simulink model "Modello_lineare_Hinfsyn"  (R2022b)
settings: Solver=VariableStepAuto  StartTime=0.0  StopTime=60  RelTol=1e-3
values from neighbouring files (symbols this model uses):
  A_tot = [A_nom B_nom*C_att ... (first row only)    [Inizializzazione_segway.m]    (also in LQG_controller.m = load("Matrici spazio di stato.mat","A_tot").A_tot; Matrici spazio di stato.mat = [0 79.8818966561 0 0 1 0 0 0 0 -0.384250591166 -200 0 ... (1)
  B_tot = [zeros(2,2); B_att]    [Inizializzazione_segway.m]    (also in LQG_controller.m = load("Matrici spazio di stato.mat","B_tot").B_tot; Matrici spazio di stato.mat = [0  0; 0  0; 894.427191  0; 0  894.427191])
  C_tot = [C_nom zeros(2,2)]    [Inizializzazione_segway.m]    (also in LQG_controller.m = load("Matrici spazio di stato.mat","C_tot").C_tot; Matrici spazio di stato.mat = [1  0  0  0; 0  1  0  0])
  D_tot = zeros(2,2)    [Inizializzazione_segway.m]    (also in LQG_controller.m = load("Matrici spazio di stato.mat","D_tot").D_tot; Matrici spazio di stato.mat = [0  0; 0  0])
undefined symbols (not defined in the file or in its folder): K_ms, K_musyn
libraries: simulink x2
settings Model: Creator=anton  LastModifiedBy=angel

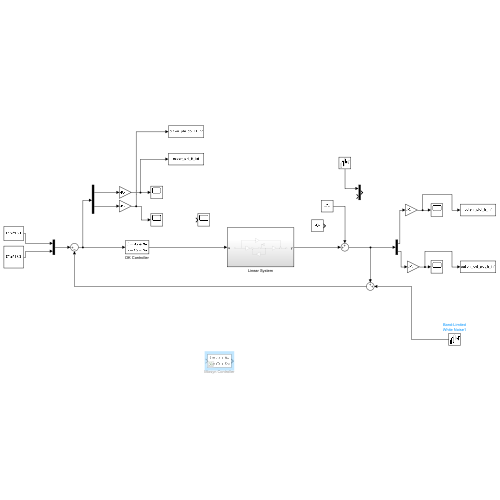
[thumbnail: Simulink's stored preview of the top-level diagram]
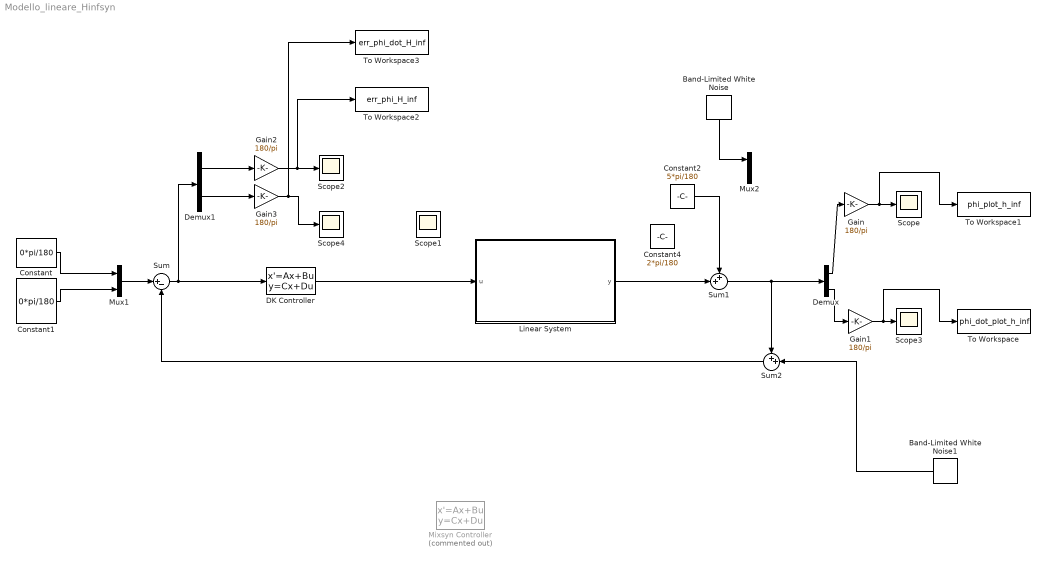
== system Modello_lineare_Hinfsyn ==
  Band-Limited White Noise : simulink/Sources/Band-Limited White Noise  Cov=[(5*pi/180)^2]  Ts=1  seed=[23341]
  Band-Limited White Noise1 : simulink/Sources/Band-Limited White Noise  Cov=[(2*pi/180)^2]  Ts=0.1  seed=[23341]
  Constant : Constant  Value=0*pi/180
  Constant1 : Constant  Value=0*pi/180
  Constant2 : Constant  Value=5*pi/180
  Constant4 : Constant  Value=2*pi/180
  DK Controller : StateSpace  A=K_musyn.A  B=K_musyn.B  C=K_musyn.C  D=K_musyn.D  InitialCondition=zeros(length(K_musyn.A),1)
  Demux : Demux  Outputs=2
  Demux1 : Demux  Outputs=2
  Gain{,1..3} (4 alike) : Gain  Gain=180/pi
  Linear System : Subsystem
  Mixsyn Controller : StateSpace  Commented=on  A=K_ms.A  B=K_ms.B  C=K_ms.C  D=K_ms.D  InitialCondition=zeros(length(K_ms.A),1)
  Mux1 : Mux  Inputs=2
  Mux2 : Mux  Inputs=2
  Scope{,1..4} (5 alike) : Scope
  Sum : Sum  Inputs=|+-
  Sum1 : Sum  Inputs=++|
  Sum2 : Sum  Inputs=++|
  To Workspace : ToWorkspace  VariableName=phi_dot_plot_h_inf  SaveFormat=Timeseries  SampleTime=-1
  To Workspace1 : ToWorkspace  VariableName=phi_plot_h_inf  SaveFormat=Timeseries  SampleTime=-1
  To Workspace2 : ToWorkspace  VariableName=err_phi_H_inf  SaveFormat=Timeseries  SampleTime=-1
  To Workspace3 : ToWorkspace  VariableName=err_phi_dot_H_inf  SaveFormat=Timeseries  SampleTime=-1
  wires:
  Sum/1 -> DK Controller/1, Demux1/1
  Constant/1 -> Mux1/1
  Mux1/1 -> Sum/1
  Constant1/1 -> Mux1/2
  Linear System/1(y) -> Sum1/2
  Sum1/1 -> Sum2/1, Demux/1
  Gain1/1 -> To Workspace/1, Scope3/1
  Demux/2 -> Gain1/1
  Demux/1 -> Gain/1
  Sum2/1 -> Sum/2
  Demux1/1 -> Gain2/1
  Gain2/1 -> To Workspace2/1, Scope2/1
  Gain3/1 -> To Workspace3/1, Scope4/1
  Demux1/2 -> Gain3/1
  Band-Limited White Noise/1 -> Mux2/1
  Constant2/1 -> Sum1/1
  Gain/1 -> To Workspace1/1, Scope/1
  DK Controller/1 -> Linear System/1(u)
  Band-Limited White Noise1/1 -> Sum2/2

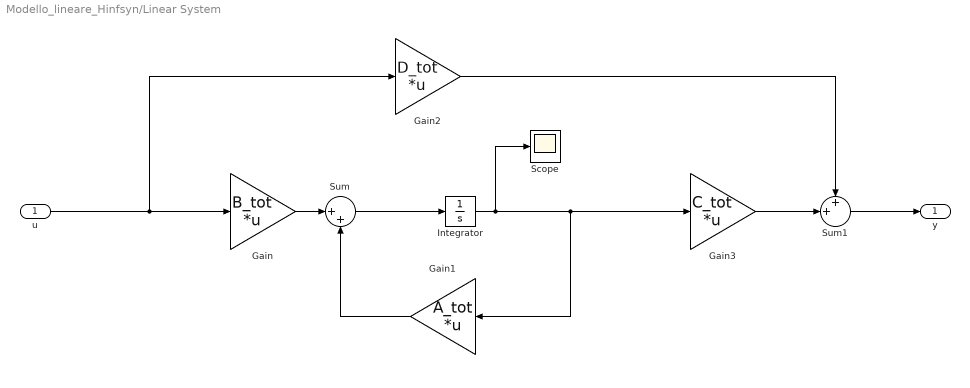
== system Modello_lineare_Hinfsyn/Linear System ==
  u : Inport
  Gain : Gain  Gain=B_tot  Multiplication=Matrix(K*u)
  Gain1 : Gain  Gain=A_tot  Multiplication=Matrix(K*u)
  Gain2 : Gain  Gain=D_tot  Multiplication=Matrix(K*u)
  Gain3 : Gain  Gain=C_tot  Multiplication=Matrix(K*u)
  Integrator : Integrator  InitialCondition=[0 0 0 0]
  Scope : Scope
  Sum : Sum  Inputs=|++
  Sum1 : Sum  Inputs=++|
  y : Outport
  wires:
  Sum/1 -> Integrator/1
  Gain1/1 -> Sum/2
  u/1 -> Gain2/1, Gain/1
  Gain3/1 -> Sum1/2
  Sum1/1 -> y/1
  Gain2/1 -> Sum1/1
  Integrator/1 -> Gain3/1, Gain1/1, Scope/1
  Gain/1 -> Sum/1
